simulink model "rangefinders_example"  (R2018b)
settings: Solver=FixedStepDiscrete  StartTime=0.0  StopTime=100  FixedStep=0.001  RelTol=1e-3
libraries: simulink x1, vrlib x1
settings Model: PacingRate=15  Creator=fabian  LastModifiedBy=fabian

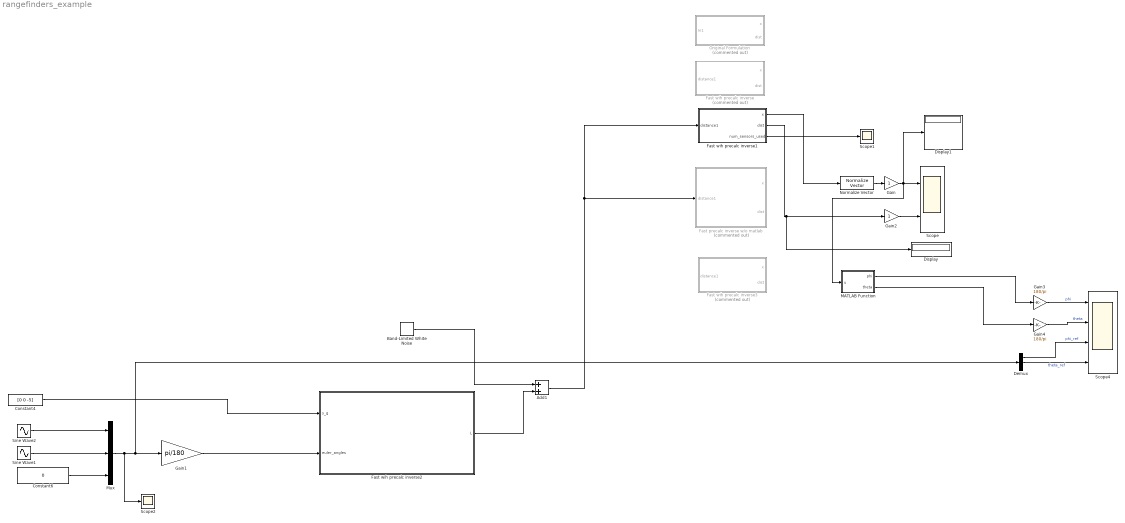
== system rangefinders_example ==
  Add1 : Sum
  Band-Limited White Noise : simulink/Sources/Band-Limited White Noise  Cov=[5e-7]  Ts=0.001  seed=[23341 14256 1236 123 5 8 4 6845 458 652 453 96 45 23341 14256 1236 123 5 8 4 6845 458 652 453 96 45]
  Constant4 : Constant  Value=[0 0 -5]  VectorParams1D=off
  Constant6 : Constant  Value=0  VectorParams1D=off
  Demux : Demux  Outputs=3
  Display : Display
  Display1 : Display
  Fast precalc inverse w/o matlab : Subsystem  Commented=on  mask{theta=[-75 -75 -75], psi=[0 90 -90]}
      mask prompts: theta "Nickwinkel"; psi "Gierwinkel"
      mask init:
      | size_n = length(theta);
      | 
      | A = zeros(size_n,3)
      | 
      | for i = 1:size_n
      |     A(i,:) = (euler2Dcm(pi/180*[0 theta(i) psi(i)])' * [1; 0; 0])';
      | end
      | 
      | A_inv = inv(A);
      | 
      | d = ones(size_n, 1)
  Fast wih precalc inverse : Subsystem  Commented=on  mask{theta=[-80 -45 -45], psi=[0 90 -90]}
      mask prompts: theta "Nickwinkel"; psi "Gierwinkel"
      mask init:
      | size_n = length(theta);
      | 
      | A = zeros(size_n,3)
      | 
      | for i = 1:size_n
      |     A(i,:) = (euler2Dcm(pi/180*[0 theta(i) psi(i)])' * [1; 0; 0])';
      | end
      | 
      | A_inv = inv(A);
      | 
      | d = ones(size_n, 1)
  Fast wih precalc inverse1 : Subsystem  mask{theta=[0:30:360, 0:30:360], psi=[repmat(0,1,13), repmat(90,1,13)]}
      mask prompts: theta "Nickwinkel"; psi "Gierwinkel"
  Fast wih precalc inverse2 : Subsystem  mask{theta=[0:30:360, 0:30:360], psi=[repmat(0,1,13), repmat(90,1,13)], range=repmat(60,1,26)}
      mask prompts: theta "Nickwinkel"; psi "Gierwinkel"
  Fast wih precalc inverse3 : Subsystem  Commented=on  mask{theta=[-75 -75 -75], psi=[0 90 -90]}
      mask prompts: theta "Nickwinkel"; psi "Gierwinkel"
  Gain : Gain
  Gain1 : Gain  Gain=pi/180
  Gain2 : Gain
  Gain3 : Gain  Gain=180/pi
  Gain4 : Gain  Gain=180/pi
  MATLAB Function : MATLAB Function  TreatAsAtomicUnit=on
  Mux : Mux  Inputs=3
  Normalize Vector : vrlib/Utilities/Normalize Vector  maxzero=0
      settings: SourceProductName=Simulink 3D Animation  SourceProductBaseCode=VR
  Original Formulation : Subsystem  Commented=on
  Scope : Scope  NumInputPorts=2
  Scope1 : Scope
  Scope2 : Scope
  Scope4 : Scope  NumInputPorts=4
  Sine Wave1 : Sin  Amplitude=60  Frequency=1/(2*pi)  SampleTime=0
  Sine Wave2 : Sin  Amplitude=170  Frequency=3.5/(2*pi)  SampleTime=0
  wires:
  Mux/1 -> Scope2/1, Demux/1, Gain1/1
  Constant6/1 -> Mux/3
  Constant4/1 -> Fast wih precalc inverse2/1(s_g)
  Gain1/1 -> Fast wih precalc inverse2/2(euler_angles)
  Gain/1 -> MATLAB Function/1(u), Display1/1, Scope/1
  Gain2/1 -> Scope/2
  Add1/1 -> Fast wih precalc inverse1/1(distance1), Fast precalc inverse w/o matlab/1(distance1)
  Normalize Vector/1 -> Gain/1
  Sine Wave1/1 -> Mux/2
  Sine Wave2/1 -> Mux/1
  MATLAB Function/1(phi) -> Gain3/1
  MATLAB Function/2(theta) -> Gain4/1
  Gain3/1 -> Scope4/1  "phi"
  Gain4/1 -> Scope4/2  "theta"
  Demux/1 -> Scope4/3  "phi_ref"
  Demux/2 -> Scope4/4  "theta_ref"
  Fast wih precalc inverse1/1(x) -> Normalize Vector/1
  Fast wih precalc inverse1/2(dist) -> Display/1, Gain2/1
  Fast wih precalc inverse2/1(L) -> Add1/2
  Fast wih precalc inverse1/3(num_sensors_used) -> Scope1/1
  Band-Limited White Noise/1 -> Add1/1

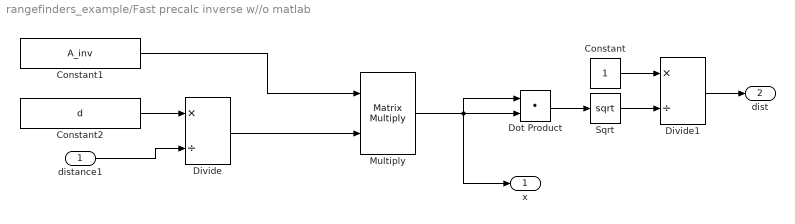
== system rangefinders_example/Fast precalc inverse w//o matlab ==
  distance1 : Inport
  Constant : Constant
  Constant1 : Constant  Value=A_inv  VectorParams1D=off
  Constant2 : Constant  Value=d  VectorParams1D=off
  Divide : Product  Inputs=*/
  Divide1 : Product  Inputs=*/
  Dot Product : DotProduct  InputSameDT=on  OutDataTypeStr=Inherit: Inherit via internal rule
  Multiply : Product  Multiplication=Matrix(*)
  Sqrt : Sqrt  SaturateOnIntegerOverflow=on
  x : Outport
  dist : Outport  Port=2
  wires:
  Constant1/1 -> Multiply/1
  Constant2/1 -> Divide/1
  distance1/1 -> Divide/2
  Divide/1 -> Multiply/2
  Multiply/1 -> Dot Product/1, x/1, Dot Product/2
  Dot Product/1 -> Sqrt/1
  Sqrt/1 -> Divide1/2
  Divide1/1 -> dist/1
  Constant/1 -> Divide1/1

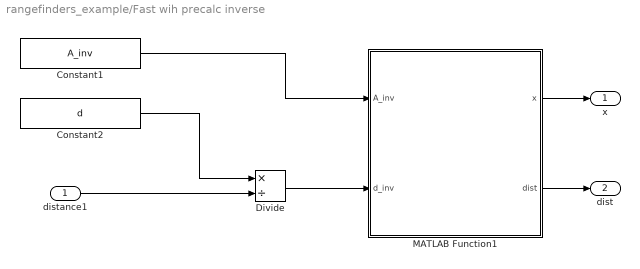
== system rangefinders_example/Fast wih precalc inverse ==
  distance1 : Inport
  Constant1 : Constant  Value=A_inv  VectorParams1D=off
  Constant2 : Constant  Value=d  VectorParams1D=off
  Divide : Product  Inputs=*/
  MATLAB Function1 : MATLAB Function  TreatAsAtomicUnit=on
  x : Outport
  dist : Outport  Port=2
  wires:
  Constant2/1 -> Divide/1
  distance1/1 -> Divide/2
  Constant1/1 -> MATLAB Function1/1(A_inv)
  Divide/1 -> MATLAB Function1/2(d_inv)
  MATLAB Function1/1(x) -> x/1
  MATLAB Function1/2(dist) -> dist/1

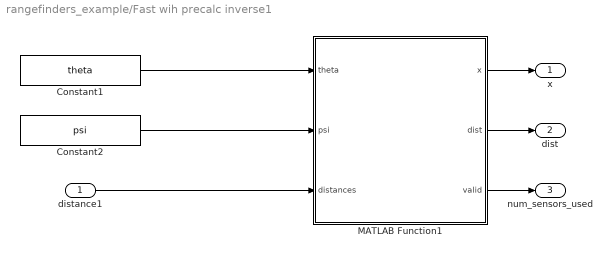
== system rangefinders_example/Fast wih precalc inverse1 ==
  distance1 : Inport
  Constant1 : Constant  Value=theta  VectorParams1D=off
  Constant2 : Constant  Value=psi  VectorParams1D=off
  MATLAB Function1 : MATLAB Function  TreatAsAtomicUnit=on
  x : Outport
  dist : Outport  Port=2
  num_sensors_used : Outport  Port=3
  wires:
  Constant1/1 -> MATLAB Function1/1(theta)
  Constant2/1 -> MATLAB Function1/2(psi)
  MATLAB Function1/1(x) -> x/1
  MATLAB Function1/2(dist) -> dist/1
  distance1/1 -> MATLAB Function1/3(distances)
  MATLAB Function1/3(valid) -> num_sensors_used/1

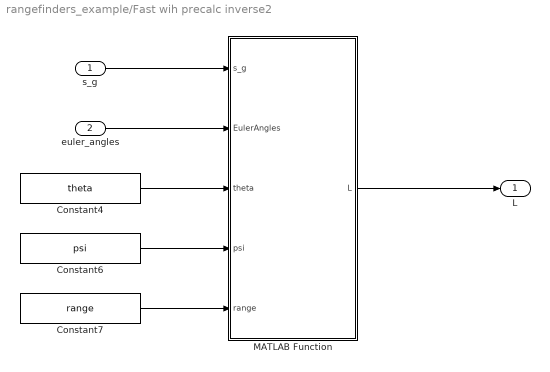
== system rangefinders_example/Fast wih precalc inverse2 ==
  s_g : Inport
  euler_angles : Inport  Port=2
  Constant4 : Constant  Value=theta  VectorParams1D=off
  Constant6 : Constant  Value=psi  VectorParams1D=off
  Constant7 : Constant  Value=range  VectorParams1D=off
  MATLAB Function : MATLAB Function  TreatAsAtomicUnit=on
  L : Outport
  wires:
  MATLAB Function/1(L) -> L/1
  Constant7/1 -> MATLAB Function/5(range)
  s_g/1 -> MATLAB Function/1(s_g)
  euler_angles/1 -> MATLAB Function/2(EulerAngles)
  Constant4/1 -> MATLAB Function/3(theta)
  Constant6/1 -> MATLAB Function/4(psi)

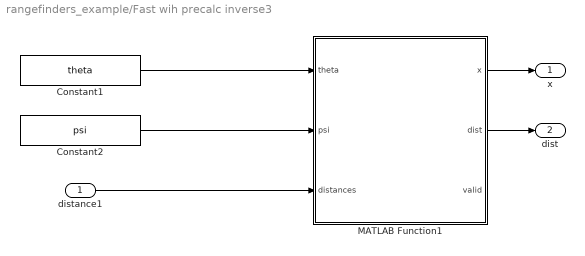
== system rangefinders_example/Fast wih precalc inverse3 ==
  distance1 : Inport
  Constant1 : Constant  Value=theta  VectorParams1D=off
  Constant2 : Constant  Value=psi  VectorParams1D=off
  MATLAB Function1 : MATLAB Function  TreatAsAtomicUnit=on
  x : Outport
  dist : Outport  Port=2
  wires:
  Constant1/1 -> MATLAB Function1/1(theta)
  Constant2/1 -> MATLAB Function1/2(psi)
  MATLAB Function1/1(x) -> x/1
  MATLAB Function1/2(dist) -> dist/1
  distance1/1 -> MATLAB Function1/3(distances)

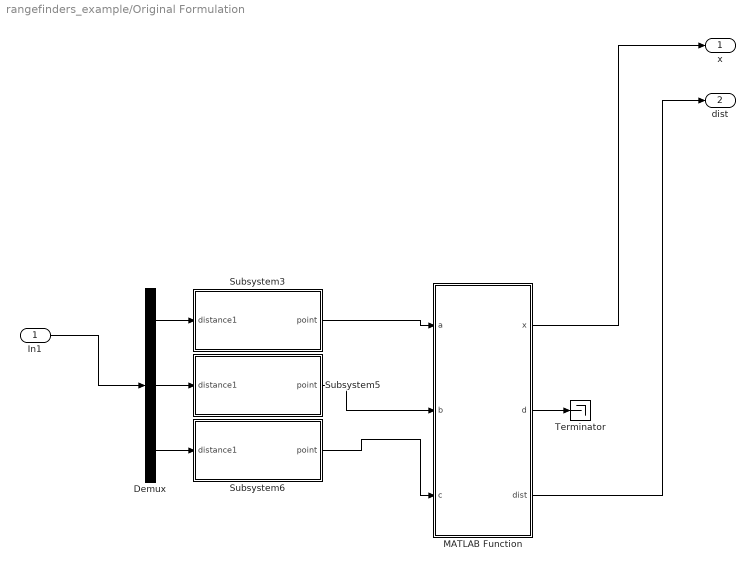
== system rangefinders_example/Original Formulation ==
  In1 : Inport
  Demux : Demux  Outputs=3
  MATLAB Function : MATLAB Function  TreatAsAtomicUnit=on
  Subsystem3 : Subsystem  mask{EulerAngles=[0 -80 0]}
      mask prompts: EulerAngles "Euler Angles"
      mask init:
      | matrix_rot_T = euler2Dcm(pi/180*EulerAngles)';
      | normal_vec = [1; 0; 0];
      | range_fnd_vec = matrix_rot_T * normal_vec;
  Subsystem5 : Subsystem  mask{EulerAngles=[0 -45 90]}
      mask prompts: EulerAngles "Euler Angles"
      mask init:
      | matrix_rot_T = euler2Dcm(pi/180*EulerAngles)';
      | normal_vec = [1; 0; 0];
      | range_fnd_vec = matrix_rot_T * normal_vec;
  Subsystem6 : Subsystem  mask{EulerAngles=[0 -45 -90]}
      mask prompts: EulerAngles "Euler Angles"
      mask init:
      | matrix_rot_T = euler2Dcm(pi/180*EulerAngles)';
      | normal_vec = [1; 0; 0];
      | range_fnd_vec = matrix_rot_T * normal_vec;
  Terminator : Terminator
  x : Outport
  dist : Outport  Port=2
  wires:
  In1/1 -> Demux/1
  Demux/2 -> Subsystem5/1(distance1)
  MATLAB Function/3(dist) -> dist/1
  MATLAB Function/1(x) -> x/1
  Demux/1 -> Subsystem3/1(distance1)
  Demux/3 -> Subsystem6/1(distance1)
  Subsystem3/1(point) -> MATLAB Function/1(a)
  Subsystem5/1(point) -> MATLAB Function/2(b)
  Subsystem6/1(point) -> MATLAB Function/3(c)
  MATLAB Function/2(d) -> Terminator/1

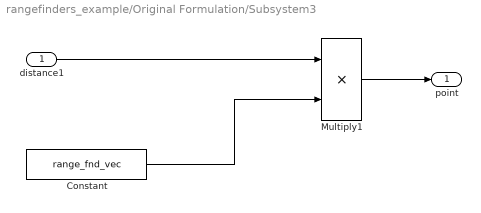
== system rangefinders_example/Original Formulation/Subsystem3 ==
  distance1 : Inport
  Constant : Constant  Value=range_fnd_vec  VectorParams1D=off
  Multiply1 : Product
  point : Outport
  wires:
  Multiply1/1 -> point/1
  Constant/1 -> Multiply1/2
  distance1/1 -> Multiply1/1

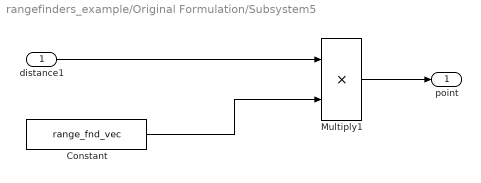
== system rangefinders_example/Original Formulation/Subsystem5 ==
  distance1 : Inport
  Constant : Constant  Value=range_fnd_vec  VectorParams1D=off
  Multiply1 : Product
  point : Outport
  wires:
  Multiply1/1 -> point/1
  Constant/1 -> Multiply1/2
  distance1/1 -> Multiply1/1

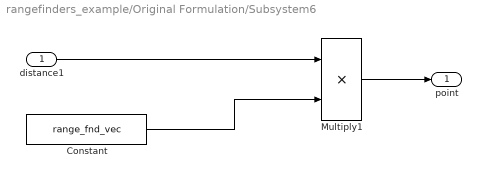
== system rangefinders_example/Original Formulation/Subsystem6 ==
  distance1 : Inport
  Constant : Constant  Value=range_fnd_vec  VectorParams1D=off
  Multiply1 : Product
  point : Outport
  wires:
  Multiply1/1 -> point/1
  Constant/1 -> Multiply1/2
  distance1/1 -> Multiply1/1

== matlab function rangefinders_example/Fast wih precalc inverse/MATLAB Function1 ==
  data: x output; A_inv input; d_inv input; dist output
function [x,dist] = fcn(A_inv,d_inv)

x = A_inv * d_inv;

dist = 1 / norm(x);

== matlab function rangefinders_example/Fast wih precalc inverse3/MATLAB Function1 ==
  data: x output; theta input; psi input; dist output; distances input; valid output
function [x,dist,valid] = fcn(theta, psi, distances)

size_n     = length(theta)+5;
size_theta = length(theta);


A = zeros(size_n, 3);

d_ones = ones(size_theta, 1);
d_inv = zeros(size_n, 1);

d_inv(1:size_theta) = d_ones ./ distances;

valid = 0;

for i = 1:size_theta
   if(distances(i) < 50)
        A(i,:) = (euler2Dcm(pi/180*[0 theta(i) psi(i)])' * [1; 0; 0])';
        valid = valid + 1;
   else
        d_inv(i) = 0;
   end
end

if(valid > 2)

    A_mat = A' * A;
    b_mat = A' * d_inv;

    x = A_mat \ b_mat;

    dist = 1 / norm(x);
else
    x = zeros(3,1);
    dist = 0;
end

== matlab function rangefinders_example/MATLAB Function ==
  data: u input; phi output; theta output
function [phi,theta] = fcn(u)

phi   = atan2(u(2), u(3));
theta = atan2(-u(1), sqrt(u(2)^2 + u(3)^2));

end

== matlab function rangefinders_example/Original Formulation/MATLAB Function ==
  data: a input; x output; b input; c input; d output; dist output
function [x,d,dist]  = fcn(a,b,c)
%ax + by + cz = d

x = zeros(3,1);

d = 1;

A = [a(1) a(2) a(3);
     b(1) b(2) b(3);
     c(1) c(2) c(3)];
 
y = [d; d; d];

x = (A'*A) \ (A'*y);
%x = A \ y;

dist = 1 / norm(x);

end

== matlab function rangefinders_example/Fast wih precalc inverse1/MATLAB Function1 ==
  data: x output; theta input; psi input; dist output; distances input; valid output
function [x,dist,valid] = fcn(theta, psi, distances)

size_n     = length(theta)+5;
size_theta = length(theta);


A = zeros(size_n, 3);

d_ones = ones(size_theta, 1);
d_inv = zeros(size_n, 1);

d_inv(1:size_theta) = d_ones ./ distances;

valid = 0;

for i = 1:size_theta
   if(distances(i) < 50)
        A(i,:) = (euler2Dcm(pi/180*[0 theta(i) psi(i)])' * [1; 0; 0])';
        valid = valid + 1;
   else
        d_inv(i) = 0;
   end
end

if(valid > 2)

    A_mat = A' * A;
    b_mat = A' * d_inv;

    x = A_mat \ b_mat;

    dist = 1 / norm(x);
else
    x = zeros(3,1);
    dist = 0;
end

== matlab function rangefinders_example/Fast wih precalc inverse2/MATLAB Function ==
  data: s_g input; EulerAngles input; theta input; psi input; L output; range input
function L  = calc_length(s_g,EulerAngles,theta,psi,range)

n  = [0 0 1];
V0 = [0 0 0];
P0 = s_g;

M_bg = euler2Dcm(EulerAngles);

L = zeros(length(theta),1);

for i=1:length(theta)
    matrix_rot_T  = euler2Dcm(pi/180*[0 theta(i) psi(i)])';
    normal_vector = matrix_rot_T * [range(i); 0; 0];
    u = (M_bg' * normal_vector)';
    [~, ~, L(i)]=plane_line_intersect(n,V0,P0,u);
end


end


function [I,check, L]=plane_line_intersect(n,V0,P0,u)
%plane_line_intersect computes the intersection of a plane and a segment(or
%a straight line)
% Inputs:
%       n: normal vector of the Plane
%       V0: any point that belongs to the Plane
%       P0: end point 1 of the segment P0P1
%       P1:  end point 2 of the segment P0P1
%
%Outputs:
%      I    is the point of interection
%     Check is an indicator:
%      0 => disjoint (no intersection)
%      1 => the plane intersects P0P1 in the unique point I
%      2 => the segment lies in the plane
%      3=>the intersection lies outside the segment P0P1
%
% Example:
% Determine the intersection of following the plane x+y+z+3=0 with the segment P0P1:
% The plane is represented by the normal vector n=[1 1 1]
% and an arbitrary point that lies on the plane, ex: V0=[1 1 -5]
% The segment is represented by the following two points
% P0=[-5 1 -1]
%P1=[1 2 3]
% [I,check]=plane_line_intersect([1 1 1],[1 1 -5],[-5 1 -1],[1 2 3]);
%This function is written by :
%                             Nassim Khaled
%                             Wayne State University
%                             Research Assistant and Phd candidate
%If you have any comments or face any problems, please feel free to leave
%your comments and i will try to reply to you as fast as possible.
L = 60;
I=[0 0 0];
P1 = P0 + u ;
w = P0 - V0;
D = dot(n,u);
N = -dot(n,w);
check=0;
if abs(D) < 10^-7        % The segment is parallel to plane
    if N == 0           % The segment lies in plane
        check=2;
        return
    else
        check=0;       %no intersection
        return
    end
end
%compute the intersection parameter
sI = N / D;
I = P0 + sI.*u;
if (sI < 0 || sI > 1)
    check= 3;          %The intersection point  lies outside the segment, so there is no intersection
    L = norm(P0-P1);
else
    L = norm(I-P0);
end

end
